simulink model "MPC_fp"  (R2016b)
settings: Solver=ode4  StartTime=0.0  StopTime=trun  FixedStep=Ts  RelTol=1e-5  EnableMultiTasking=on
undefined symbols (not defined in the file): Ainq_mpc, binq_mpc, H2_x0_mpc, H3_mpc, N_mpc, Nx, PLANT, ref_f, slr, Ts, uss_0, uss_f, x0
settings Model: Creator=arnold  LastModifiedBy=arnold
settings DataIOCC: SaveFormat=Array  SaveOutput=off  SaveState=on  InspectSignalLogs=on  TimeSaveName=tout_ptos
settings OptimizationCC: LifeSpan=inf
settings DebuggingCC: SolverPrmCheckMsg=warning  SFUnexpectedBacktrackingDiag=warning  SFNoUnconditionalDefaultTransitionDiag=warning  SFExecutionAtInitializationDiag=none
settings HardwareCC: ProdBitPerPointer=32  ProdBitPerSizeT=32  ProdBitPerPtrDiffT=32  ProdLargestAtomicFloat=None  ProdIntDivRoundTo=Undefined  ProdEndianess=Unspecified  ProdWordSize=32  ProdHWDeviceType=32-bit Generic
settings ModelReferenceCC: PropagateSignalLabelsOutOfModel=off
settings GRTTargetCC: TargetLangStandard=C89/C90 (ANSI)  GeneratePreprocessorConditionals=Disable all
settings ConfigComp: CovMetricSettings=dw  CovHtmlReporting=on  CovSaveCumulativeToWorkspaceVar=on  CovSaveSingleToWorkspaceVar=on  CovExternalEMLEnable=off  CovSFcnEnable=off

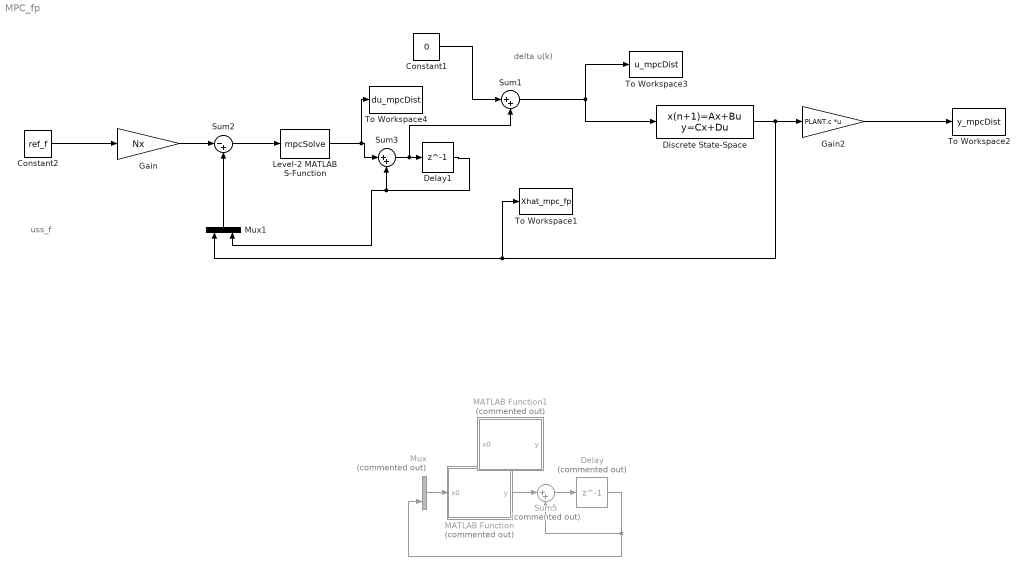
== system MPC_fp ==
  note: uss_f
  note: delta u(k)
  Constant1 : Constant  Value=0
  Constant2 : Constant  Value=ref_f
  Delay : Delay  Commented=on  DelayLength=1  InitialCondition=uss_0-uss_f  SampleTime=Ts
  Delay1 : Delay  DelayLength=1  InitialCondition=uss_0  SampleTime=Ts
  Discrete State-Space : DiscreteStateSpace  A=PLANT.a  B=PLANT.b  C=eye(size(PLANT.b,1))  D=zeros(size(PLANT.b,1),1)  X0=x0  SampleTime=Ts
  Gain : Gain  Gain=Nx
  Gain2 : Gain  Gain=PLANT.c  Multiplication=Matrix(K*u)
  Level-2 MATLAB S-Function : M-S-Function  FunctionName=mpcSolve  Parameters=mpcProb1
  MATLAB Function : MATLAB Function  Commented=on  TreatAsAtomicUnit=on
  MATLAB Function1 : MATLAB Function  Commented=on  TreatAsAtomicUnit=on
  Mux : Mux  Commented=on  Inputs=2
  Mux1 : Mux  Inputs=2
  Sum1 : Sum  Inputs=|++
  Sum2 : Sum  Inputs=|-+
  Sum3 : Sum  Inputs=|++
  Sum5 : Sum  Commented=on  Inputs=|++
  To Workspace1 : ToWorkspace  VariableName=Xhat_mpc_fp  SaveFormat=Timeseries  SampleTime=-1
      settings: Save2DSignal=2-D array (concatenate along first dimension)
  To Workspace2 : ToWorkspace  VariableName=y_mpcDist  SaveFormat=Timeseries  SampleTime=-1
      settings: Save2DSignal=2-D array (concatenate along first dimension)
  To Workspace3 : ToWorkspace  VariableName=u_mpcDist  SaveFormat=Timeseries  SampleTime=-1
      settings: Save2DSignal=2-D array (concatenate along first dimension)
  To Workspace4 : ToWorkspace  VariableName=du_mpcDist  SaveFormat=Timeseries  SampleTime=-1
      settings: Save2DSignal=2-D array (concatenate along first dimension)
  wires:
  Gain/1 -> Sum2/1
  Sum1/1 -> Discrete State-Space/1, To Workspace3/1
  Discrete State-Space/1 -> Mux1/1, To Workspace1/1, Gain2/1
  Gain2/1 -> To Workspace2/1
  Mux/1 -> MATLAB Function/1(x0)
  Delay/1 -> Mux/2, Sum5/2
  Sum5/1 -> Delay/1
  MATLAB Function/1(y) -> Sum5/1
  Sum2/1 -> Level-2 MATLAB S-Function/1
  Delay1/1 -> Mux1/2, Sum3/2
  Sum3/1 -> Sum1/2, Delay1/1
  Constant2/1 -> Gain/1
  Mux1/1 -> Sum2/2
  Level-2 MATLAB S-Function/1 -> To Workspace4/1, Sum3/1
  Constant1/1 -> Sum1/1

== matlab function MPC_fp/MATLAB Function1 ==
  data: x0 input size=Ns_mpc; y output; H3_mpc parameter; H2_x0_mpc parameter; Ainq_mpc parameter; binq_mpc parameter; N_mpc parameter; slr parameter
function y = fcn(x0, H3_mpc, H2_x0_mpc, Ainq_mpc, binq_mpc, N_mpc, slr)
coder.extrinsic('keyboard');
coder.extrinsic('lqrMPCSolve');

assert(N_mpc<128)
% H2 = 2*x0'*G'*W1*H - 2*Req'*W1*H - 2*Ueq'*W2;
% x_0 = [uk_m1; x0];
H2_mpc = (H2_x0_mpc*x0);

% Ainq_mpc = [1, zeros(1,N_mpc-1);
%             -1, zeros(1,N_mpc-1);
%             Ainq_mpc];
% binq_mpc = [slr+uk_m1;
%             slr-uk_m1;
%             binq_mpc];
        
u = zeros(N_mpc,1);
u = lqrMPCSolve(H3_mpc, H2_mpc, Ainq_mpc, binq_mpc);
% keyboard



y = u(1);

== matlab function MPC_fp/MATLAB Function ==
  data: x0 input size=Ns_recyc; y output; H3_mpc parameter; H2_x0_mpc parameter; Ainq_mpc parameter; binq_mpc parameter; N_mpc parameter
function y = fcn(x0, H3_mpc, H2_x0_mpc, Ainq_mpc, binq_mpc, N_mpc)
coder.extrinsic('keyboard');
coder.extrinsic('lqrMPCSolve');

assert(N_mpc<128)
% H2 = 2*x0'*G'*W1*H - 2*Req'*W1*H - 2*Ueq'*W2;
H2_mpc = (H2_x0_mpc*x0);


u = zeros(N_mpc,1);
u = lqrMPCSolve(H3_mpc, H2_mpc, Ainq_mpc, binq_mpc);
% keyboard



y = u(1);
